simulink model "LiderSeguidor"  (R2021a)
settings: Solver=VariableStepAuto  StartTime=0.0  StopTime=inf  RelTol=1e-3
libraries: robotlib x5
settings Model: Creator=julio  LastModifiedBy=julio

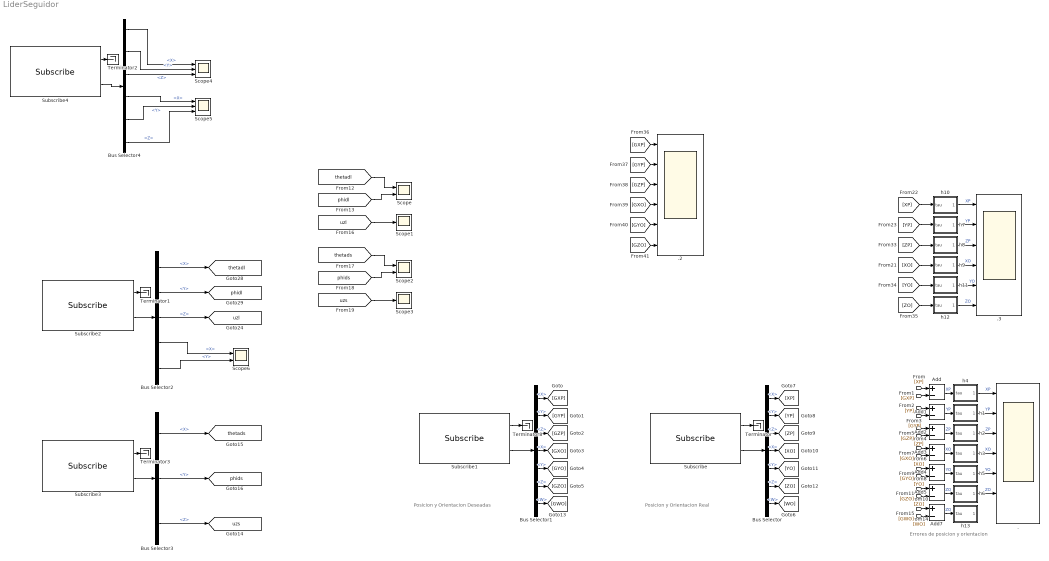
== system LiderSeguidor ==
  note: Posicion y Orientacion Real
  note: Errores de posicion y orientacion
  note: Posicion y Orientacion Deseadas
  . : Scope  NumInputPorts=7
  .2 : Scope  NumInputPorts=6
  .3 : Scope  NumInputPorts=6
  Add{,1..5,7} (7 alike) : Sum  Inputs=+-
  Bus Selector : BusSelector  OutputSignals=Pose.Position.X,Pose.Position.Y,Pose.Position.Z,Pose.Orientation.X,Pose.Orientation.Y,Pose.Orientation.Z,Pose.Orientation.W
  Bus Selector1 : BusSelector  OutputSignals=Pose.Position.X,Pose.Position.Y,Pose.Position.Z,Pose.Orientation.X,Pose.Orientation.Y,Pose.Orientation.Z,Pose.Orientation.W
  Bus Selector2 : BusSelector  OutputSignals=Linear.X,Linear.Y,Linear.Z,Angular.X,Angular.Y
  Bus Selector3 : BusSelector  OutputSignals=Linear.X,Linear.Y,Linear.Z
  Bus Selector4 : BusSelector  OutputSignals=Linear.X,Linear.Y,Linear.Z,Angular.X,Angular.Y,Angular.Z
  Scope : Scope  NumInputPorts=2
  Scope1 : Scope
  Scope2 : Scope  NumInputPorts=2
  Scope3 : Scope
  Scope4 : Scope  NumInputPorts=3
  Scope5 : Scope  NumInputPorts=3
  Scope6 : Scope  NumInputPorts=2
  Subscribe : robotlib/Subscribe  topicSource=Select from ROS network  topic=/crazyflie/vrpn_client_node/crazyflie/pose  messageType=geometry_msgs/PoseStamped  SampleTime=-1  legacyBusStruct=off  messageQueueLength=1
  Subscribe1 : robotlib/Subscribe  topicSource=Select from ROS network  topic=/crazyflie/goal  messageType=geometry_msgs/PoseStamped  SampleTime=-1  legacyBusStruct=off  messageQueueLength=1
  Subscribe2 : robotlib/Subscribe  topicSource=Select from ROS network  topic=/crazyflie1/cmd_vel  messageType=geometry_msgs/Twist  SampleTime=-1  legacyBusStruct=off  messageQueueLength=1
  Subscribe3 : robotlib/Subscribe  topicSource=Select from ROS network  topic=/crazyflie2/cmd_vel  messageType=geometry_msgs/Twist  SampleTime=-1  legacyBusStruct=off  messageQueueLength=1
  Subscribe4 : robotlib/Subscribe  topicSource=Select from ROS network  topic=/crazyflie2/info_leader  messageType=geometry_msgs/Twist  SampleTime=-1  legacyBusStruct=off  messageQueueLength=1
  Terminator{,1..3,8} (5 alike) : Terminator
  h1 : Subsystem
  h10 : Subsystem
  h11 : Subsystem
  h12 : Subsystem
  h13 : Subsystem
  h2 : Subsystem
  h3 : Subsystem
  h4 : Subsystem
  h5 : Subsystem
  h6 : Subsystem
  h7 : Subsystem
  h8 : Subsystem
  h9 : Subsystem
  tag scope: phidl=global, phids=global, thetadl=global, thetads=global, uzl=global, uzs=global
  wires:
  [GXP] -> .2/1
  Subscribe1/1 -> Terminator8/1
  h6/1(Out1) -> ./6  "ZO"
  h1/1(Out1) -> ./2  "YP"
  h3/1(Out1) -> ./4  "XO"
  h4/1(Out1) -> ./1  "XP"
  h12/1(Out1) -> .3/6  "ZO"
  h5/1(Out1) -> ./5  "YO"
  h2/1(Out1) -> ./3  "ZP"
  Add3/1 -> h3/1(tau)  "XO"
  [GYO] -> .2/5
  [GXO] -> .2/4
  Bus Selector1/7 -> [GWO]  "<W>"
  Subscribe2/1 -> Terminator1/1
  h9/1(Out1) -> .3/4  "XO"
  Subscribe2/2 -> Bus Selector2/1
  [YP] -> Add1/1
  [GYP] -> Add1/2
  [GXP] -> Add/2
  Bus Selector1/3 -> [GZP]  "<Z>"
  h10/1(Out1) -> .3/1  "XP"
  Add1/1 -> h1/1(tau)  "YP"
  Add2/1 -> h2/1(tau)  "ZP"
  [GZO] -> Add5/2
  [XO] -> h9/1(tau)
  Bus Selector1/5 -> [GYO]  "<Y>"
  Add5/1 -> h6/1(tau)  "ZO"
  [ZO] -> Add5/1
  [XP] -> Add/1
  Add4/1 -> h5/1(tau)  "YO"
  [GZP] -> .2/3
  [YO] -> h11/1(tau)
  Bus Selector/1 -> [XP]  "<X>"
  [YP] -> h7/1(tau)
  Bus Selector/5 -> [YO]  "<Y>"
  Bus Selector/6 -> [ZO]  "<Z>"
  Add/1 -> h4/1(tau)  "XP"
  Bus Selector1/1 -> [GXP]  "<X>"
  Bus Selector2/3 -> [uzl]  "<Z>"
  Bus Selector1/6 -> [GZO]  "<Z>"
  Subscribe1/2 -> Bus Selector1/1
  Bus Selector/3 -> [ZP]  "<Z>"
  h7/1(Out1) -> .3/2  "YP"
  [YO] -> Add4/1
  Bus Selector/2 -> [YP]  "<Y>"
  [GXO] -> Add3/2
  Bus Selector/4 -> [XO]  "<X>"
  [ZP] -> h8/1(tau)
  Bus Selector1/2 -> [GYP]  "<Y>"
  Subscribe/1 -> Terminator/1
  [XP] -> h10/1(tau)
  Bus Selector2/1 -> [thetadl]  "<X>"
  h8/1(Out1) -> .3/3  "ZP"
  [WO] -> Add7/1
  [GZP] -> Add2/2
  h11/1(Out1) -> .3/5  "YO"
  Bus Selector2/2 -> [phidl]  "<Y>"
  [XO] -> Add3/1
  Bus Selector/7 -> [WO]  "<W>"
  [ZO] -> h12/1(tau)
  [GWO] -> Add7/2
  Subscribe/2 -> Bus Selector/1
  [GYP] -> .2/2
  [GZO] -> .2/6
  [GYO] -> Add4/2
  Bus Selector1/4 -> [GXO]  "<X>"
  Add7/1 -> h13/1(tau)  "ZO"
  [ZP] -> Add2/1
  Subscribe3/2 -> Bus Selector3/1
  Bus Selector3/3 -> [uzs]  "<Z>"
  Subscribe3/1 -> Terminator3/1
  Bus Selector3/2 -> [phids]  "<Y>"
  Bus Selector3/1 -> [thetads]  "<X>"
  [thetadl] -> Scope/1
  [phidl] -> Scope/2
  [uzl] -> Scope1/1
  [thetads] -> Scope2/1
  [uzs] -> Scope3/1
  [phids] -> Scope2/2
  Subscribe4/2 -> Bus Selector4/1
  Bus Selector4/3 -> Scope4/3  "<Z>"
  Subscribe4/1 -> Terminator2/1
  Bus Selector4/2 -> Scope4/2  "<Y>"
  Bus Selector4/1 -> Scope4/1  "<X>"
  Bus Selector4/4 -> Scope5/1  "<X>"
  Bus Selector4/5 -> Scope5/2  "<Y>"
  Bus Selector4/6 -> Scope5/3  "<Z>"
  Bus Selector2/4 -> Scope6/1  "<X>"
  Bus Selector2/5 -> Scope6/2  "<Y>"

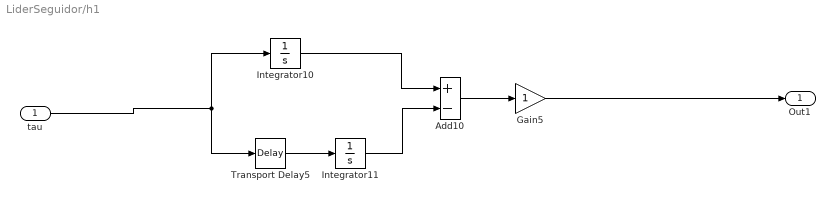
== system LiderSeguidor/h1 ==
  tau : Inport
  Add10 : Sum  Inputs=+-
  Gain5 : Gain
  Integrator10 : Integrator
  Integrator11 : Integrator
  Transport Delay5 : TransportDelay  BufferSize=2048
  Out1 : Outport  VectorParamsAs1DForOutWhenUnconnected=off
  wires:
  Add10/1 -> Gain5/1
  Gain5/1 -> Out1/1
  Integrator11/1 -> Add10/2
  Integrator10/1 -> Add10/1
  Transport Delay5/1 -> Integrator11/1
  tau/1 -> Transport Delay5/1, Integrator10/1

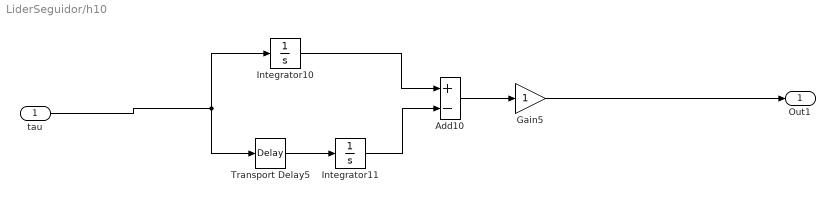
== system LiderSeguidor/h10 ==
  tau : Inport
  Add10 : Sum  Inputs=+-
  Gain5 : Gain
  Integrator10 : Integrator
  Integrator11 : Integrator
  Transport Delay5 : TransportDelay  BufferSize=2048
  Out1 : Outport  VectorParamsAs1DForOutWhenUnconnected=off
  wires:
  Add10/1 -> Gain5/1
  Gain5/1 -> Out1/1
  Integrator11/1 -> Add10/2
  Integrator10/1 -> Add10/1
  Transport Delay5/1 -> Integrator11/1
  tau/1 -> Transport Delay5/1, Integrator10/1

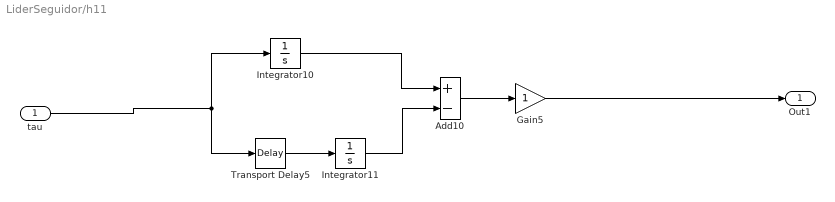
== system LiderSeguidor/h11 ==
  tau : Inport
  Add10 : Sum  Inputs=+-
  Gain5 : Gain
  Integrator10 : Integrator
  Integrator11 : Integrator
  Transport Delay5 : TransportDelay  BufferSize=2048
  Out1 : Outport  VectorParamsAs1DForOutWhenUnconnected=off
  wires:
  Add10/1 -> Gain5/1
  Gain5/1 -> Out1/1
  Integrator11/1 -> Add10/2
  Integrator10/1 -> Add10/1
  Transport Delay5/1 -> Integrator11/1
  tau/1 -> Transport Delay5/1, Integrator10/1

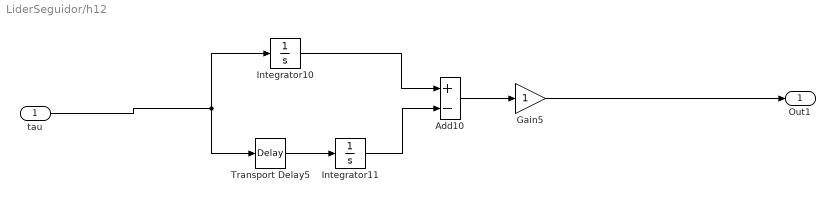
== system LiderSeguidor/h12 ==
  tau : Inport
  Add10 : Sum  Inputs=+-
  Gain5 : Gain
  Integrator10 : Integrator
  Integrator11 : Integrator
  Transport Delay5 : TransportDelay  BufferSize=2048
  Out1 : Outport  VectorParamsAs1DForOutWhenUnconnected=off
  wires:
  tau/1 -> Integrator10/1, Transport Delay5/1
  Transport Delay5/1 -> Integrator11/1
  Integrator10/1 -> Add10/1
  Integrator11/1 -> Add10/2
  Gain5/1 -> Out1/1
  Add10/1 -> Gain5/1

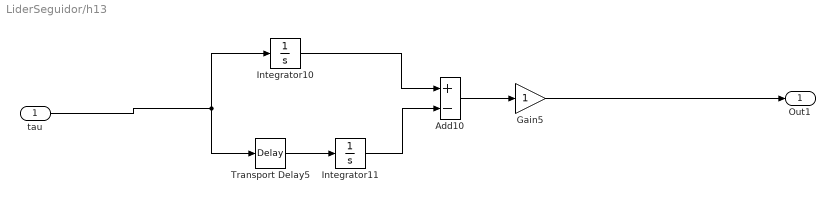
== system LiderSeguidor/h13 ==
  tau : Inport
  Add10 : Sum  Inputs=+-
  Gain5 : Gain
  Integrator10 : Integrator
  Integrator11 : Integrator
  Transport Delay5 : TransportDelay  BufferSize=2048
  Out1 : Outport  VectorParamsAs1DForOutWhenUnconnected=off
  wires:
  Add10/1 -> Gain5/1
  Gain5/1 -> Out1/1
  Integrator11/1 -> Add10/2
  Integrator10/1 -> Add10/1
  Transport Delay5/1 -> Integrator11/1
  tau/1 -> Transport Delay5/1, Integrator10/1

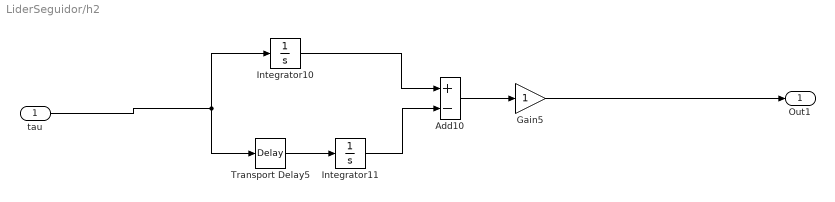
== system LiderSeguidor/h2 ==
  tau : Inport
  Add10 : Sum  Inputs=+-
  Gain5 : Gain
  Integrator10 : Integrator
  Integrator11 : Integrator
  Transport Delay5 : TransportDelay  BufferSize=2048
  Out1 : Outport  VectorParamsAs1DForOutWhenUnconnected=off
  wires:
  tau/1 -> Integrator10/1, Transport Delay5/1
  Transport Delay5/1 -> Integrator11/1
  Integrator10/1 -> Add10/1
  Integrator11/1 -> Add10/2
  Gain5/1 -> Out1/1
  Add10/1 -> Gain5/1

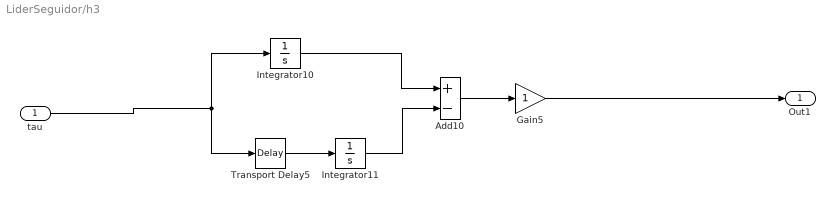
== system LiderSeguidor/h3 ==
  tau : Inport
  Add10 : Sum  Inputs=+-
  Gain5 : Gain
  Integrator10 : Integrator
  Integrator11 : Integrator
  Transport Delay5 : TransportDelay  BufferSize=2048
  Out1 : Outport  VectorParamsAs1DForOutWhenUnconnected=off
  wires:
  Add10/1 -> Gain5/1
  Gain5/1 -> Out1/1
  Integrator11/1 -> Add10/2
  Integrator10/1 -> Add10/1
  Transport Delay5/1 -> Integrator11/1
  tau/1 -> Transport Delay5/1, Integrator10/1

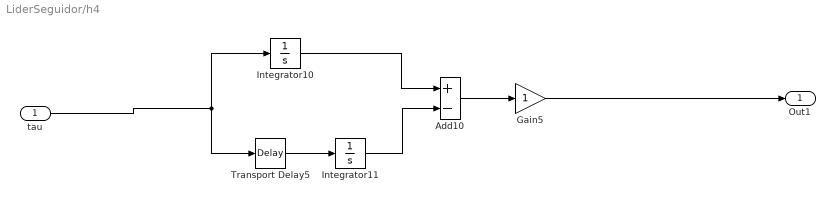
== system LiderSeguidor/h4 ==
  tau : Inport
  Add10 : Sum  Inputs=+-
  Gain5 : Gain
  Integrator10 : Integrator
  Integrator11 : Integrator
  Transport Delay5 : TransportDelay  BufferSize=2048
  Out1 : Outport  VectorParamsAs1DForOutWhenUnconnected=off
  wires:
  tau/1 -> Integrator10/1, Transport Delay5/1
  Transport Delay5/1 -> Integrator11/1
  Integrator10/1 -> Add10/1
  Integrator11/1 -> Add10/2
  Gain5/1 -> Out1/1
  Add10/1 -> Gain5/1

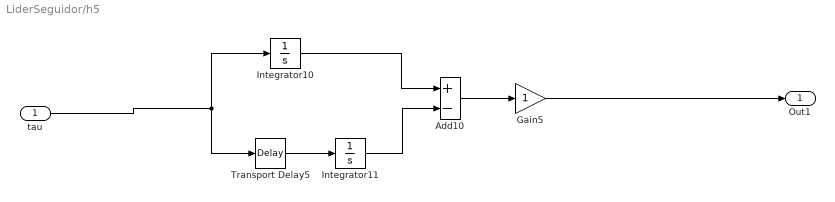
== system LiderSeguidor/h5 ==
  tau : Inport
  Add10 : Sum  Inputs=+-
  Gain5 : Gain
  Integrator10 : Integrator
  Integrator11 : Integrator
  Transport Delay5 : TransportDelay  BufferSize=2048
  Out1 : Outport  VectorParamsAs1DForOutWhenUnconnected=off
  wires:
  tau/1 -> Integrator10/1, Transport Delay5/1
  Transport Delay5/1 -> Integrator11/1
  Integrator10/1 -> Add10/1
  Integrator11/1 -> Add10/2
  Gain5/1 -> Out1/1
  Add10/1 -> Gain5/1

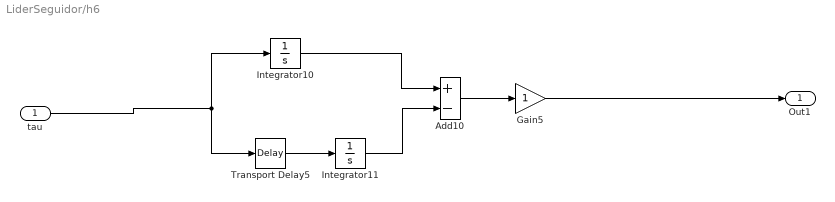
== system LiderSeguidor/h6 ==
  tau : Inport
  Add10 : Sum  Inputs=+-
  Gain5 : Gain
  Integrator10 : Integrator
  Integrator11 : Integrator
  Transport Delay5 : TransportDelay  BufferSize=2048
  Out1 : Outport  VectorParamsAs1DForOutWhenUnconnected=off
  wires:
  Add10/1 -> Gain5/1
  Gain5/1 -> Out1/1
  Integrator11/1 -> Add10/2
  Integrator10/1 -> Add10/1
  Transport Delay5/1 -> Integrator11/1
  tau/1 -> Transport Delay5/1, Integrator10/1

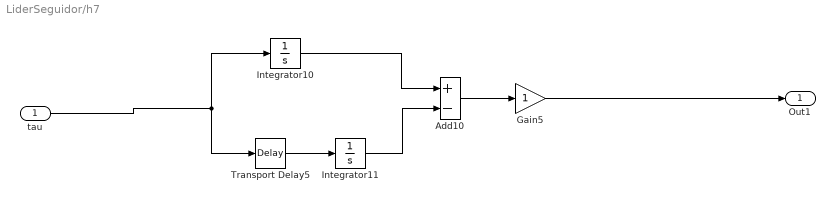
== system LiderSeguidor/h7 ==
  tau : Inport
  Add10 : Sum  Inputs=+-
  Gain5 : Gain
  Integrator10 : Integrator
  Integrator11 : Integrator
  Transport Delay5 : TransportDelay  BufferSize=2048
  Out1 : Outport  VectorParamsAs1DForOutWhenUnconnected=off
  wires:
  tau/1 -> Integrator10/1, Transport Delay5/1
  Transport Delay5/1 -> Integrator11/1
  Integrator10/1 -> Add10/1
  Integrator11/1 -> Add10/2
  Gain5/1 -> Out1/1
  Add10/1 -> Gain5/1

== system LiderSeguidor/h8 ==
  tau : Inport
  Add10 : Sum  Inputs=+-
  Gain5 : Gain
  Integrator10 : Integrator
  Integrator11 : Integrator
  Transport Delay5 : TransportDelay  BufferSize=2048
  Out1 : Outport  VectorParamsAs1DForOutWhenUnconnected=off
  wires:
  Add10/1 -> Gain5/1
  Gain5/1 -> Out1/1
  Integrator11/1 -> Add10/2
  Integrator10/1 -> Add10/1
  Transport Delay5/1 -> Integrator11/1
  tau/1 -> Transport Delay5/1, Integrator10/1

== system LiderSeguidor/h9 ==
  tau : Inport
  Add10 : Sum  Inputs=+-
  Gain5 : Gain
  Integrator10 : Integrator
  Integrator11 : Integrator
  Transport Delay5 : TransportDelay  BufferSize=2048
  Out1 : Outport  VectorParamsAs1DForOutWhenUnconnected=off
  wires:
  tau/1 -> Integrator10/1, Transport Delay5/1
  Transport Delay5/1 -> Integrator11/1
  Integrator10/1 -> Add10/1
  Integrator11/1 -> Add10/2
  Gain5/1 -> Out1/1
  Add10/1 -> Gain5/1
